simulink model "Lab0"  (R2014a)
settings: Solver=FixedStepDiscrete  StartTime=0.0  StopTime=15  FixedStep=.001  RelTol=1e-3
libraries: embdlinuxlib x1, dspswit3 x1, dspbuff3 x1, dspsigops x1
settings Model: SimulationMode=external  ExtModeTrigDuration=100  Creator=Becky  LastModifiedBy=reck2
settings OptimizationCC: OptimizeModelRefInitCode=on  LifeSpan=1
settings DebuggingCC: UnderspecifiedInitializationDetection=Classic  SolverPrmCheckMsg=none
settings HardwareCC: ProdLargestAtomicInteger=Long  ProdLargestAtomicFloat=Double  ProdEndianess=LittleEndian  ProdHWDeviceType=ARM Compatible->ARM Cortex
settings RTWCC: SystemTargetFile=realtime.tlc  GenerateMakefile=off  TemplateMakefile=realtime.tmf  Description=Run on Target Hardware  RTWVerbose=off  ProcessScript=realtime_make_rtw_hook
settings STFCustomTargetCC: TargetLibSuffix=.a  GenerateSampleERTMain=on  ConcurrentExecutionCompliant=off  GeneratePreprocessorConditionals=Use local settings  ERTCustomFileBanners=on  SupportNonInlinedSFcns=off  SupportVariableSizeSignals=on  MATLABClassNameForMDSCustomization=Simulink.SoftwareTarget.ERTCustomization  GRTInterface=off  SystemTargetFile=realtime.tlc
settings ERTTargetCC: CombineOutputUpdateFcns=off  SupportContinuousTime=on  SupportVariableSizeSignals=on  ExtModeMexArgs='192.168.0.3' 0 17725  ERTSrcFileBannerTemplate=realtime_code_template.cgt  ERTHdrFileBannerTemplate=realtime_code_template.cgt  ERTDataSrcFileTemplate=realtime_code_template.cgt  ERTDataHdrFileTemplate=realtime_code_template.cgt  ERTCustomFileTemplate=realtime_file_process.tlc

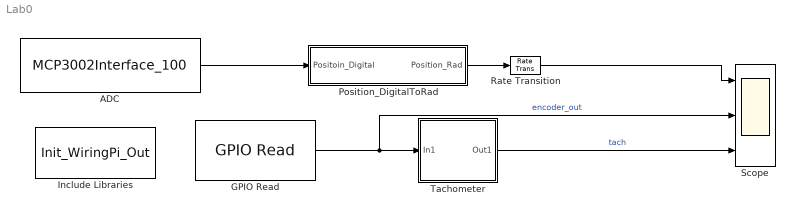
== system Lab0 ==
  ADC : S-Function  InitFcn=try, set_param(gcb,'FunctionName','MCP3002Interface_100'), end  FunctionName=MCP3002Interface_100  SFunctionModules=MCP3002Interface_100_wrapper  EnableBusSupport=off  mask(S-Function Builder){}
      mask help: Simulink:masks:SFunctionBuilder_MD
      mask init:
      | val = [[.9  0.75 0.75 1 1 .9 .9 1]',[1 1 0.75 0.75 .9 .9 1 .9]'];try , sys = get_param(gcb,'SfunBuilderFcnName');if isempty(sys), sys = get_param(gcb,'FunctionName'); end,catch, sys = get_param(gcb,'FunctionName'); end
      settings: CopyFcn=set_param(gcbh,'LinkStatus','none')  PreSaveFcn=try, set_param(gcb,'FunctionName','MCP3002Interface_100'), end  OpenFcn=sfunctionwizard(gcbh)
      mask Display: plot(val(:,1),val(:,2)),disp(sys), port_label('output',1,'y0')
  GPIO Read : embdlinuxlib/GPIO Read  board=Model B Rev2  gpio=22  internalResistor=Off  sampleTime=0.001  direction=Input  blockPlatform=Raspberry Pi
  Include Libraries : S-Function  InitFcn=try, set_param(gcb,'FunctionName','Init_WiringPi_Out'), end  FunctionName=Init_WiringPi_Out  Parameters=uint8(0),uint8(7)  SFunctionModules=Init_WiringPi_Out_wrapper  EnableBusSupport=off  mask(S-Function Builder){}
      mask init: same as Lab0/ADC
      settings: CopyFcn=set_param(gcbh,'LinkStatus','none')  PreSaveFcn=try, set_param(gcb,'FunctionName','Init_WiringPi_Out'), end  OpenFcn=sfunctionwizard(gcbh)
      mask Display: plot(val(:,1),val(:,2)),disp(sys)
  Position_DigitalToRad : Subsystem
  Rate Transition : RateTransition
  Scope : Scope  NumInputPorts=3
      settings: TimeRange=15  YMin=0~-0.2~0  YMax=6.5~1.2~100
  Tachometer : Subsystem
  wires:
  GPIO Read/1 -> Tachometer/1(In1), Scope/2  "encoder_out"
  Tachometer/1(Out1) -> Scope/3  "tach"
  ADC/1 -> Position_DigitalToRad/1(Positoin_Digital)
  Position_DigitalToRad/1(Position_Rad) -> Rate Transition/1
  Rate Transition/1 -> Scope/1

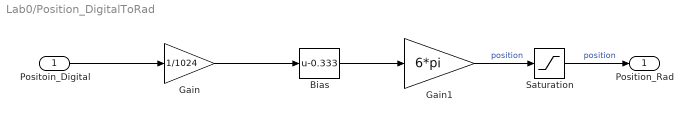
== system Lab0/Position_DigitalToRad ==
  Positoin_Digital : Inport
  Bias : Bias  Bias=-0.333
  Gain : Gain  Gain=1/1024
  Gain1 : Gain  Gain=6*pi
  Saturation : Saturate  UpperLimit=2*pi+.3  LowerLimit=0
  Position_Rad : Outport
  wires:
  Gain/1 -> Bias/1
  Bias/1 -> Gain1/1
  Gain1/1 -> Saturation/1  "position"
  Saturation/1 -> Position_Rad/1  "position"
  Positoin_Digital/1 -> Gain/1

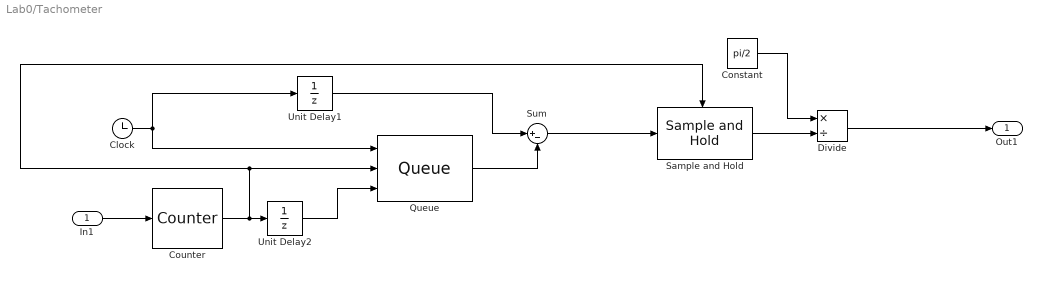
== system Lab0/Tachometer ==
  In1 : Inport
  Clock : Clock
      settings: Decimation=1000
  Constant : Constant  Value=pi/2
  Counter : dspswit3/Counter  Direction=Up  CountEvent=Rising edge  CounterSize=User defined  MaxCount=4  InitialCount=0  Output=Hit  HitValue=1  ResetInput=off  SamplesPerFrame=1  Ts=1  CntDtype=double  HitDtype=Logical
  Divide : Product  Inputs=*/
  Queue : dspbuff3/Queue  depth=2  trigger=Rising edge  overflow=Ignore  pes=Warning  eso=off  fso=off  nso=off  clr=off  clrOutport=off  adf=on
  Sample and Hold : dspsigops/Sample and Hold  trig=Rising edge  initCond=1  latchinput=off
  Sum : Sum  Inputs=|+-
  Unit Delay1 : UnitDelay  SampleTime=-1
  Unit Delay2 : UnitDelay  SampleTime=-1
  Out1 : Outport
  wires:
  In1/1 -> Counter/1
  Queue/1 -> Sum/2
  Clock/1 -> Unit Delay1/1, Queue/1
  Sum/1 -> Sample and Hold/1
  Sample and Hold/1 -> Divide/2
  Constant/1 -> Divide/1
  Divide/1 -> Out1/1
  Counter/1 -> Sample and Hold/Trigger, Queue/2, Unit Delay2/1
  Unit Delay2/1 -> Queue/3
  Unit Delay1/1 -> Sum/1
